simulink model "Pole_placement_track"  (R2023b)
settings: Solver=VariableStepAuto  StartTime=0.0  StopTime=50.0  RelTol=1e-3
values from neighbouring files (symbols this model uses):
  A = double(A)    [Rotational_inverted_pendulum.m]
  A_uns = double(A_uns)    [Rotational_inverted_pendulum.m]
  B = double(B)    [Rotational_inverted_pendulum.m]
  B_uns = double(B_uns)    [Rotational_inverted_pendulum.m]
  C = [1 0 0 0 ... (first row only)    [Rotational_inverted_pendulum.m]
  D = [0 ... (first row only)    [Rotational_inverted_pendulum.m]
  K_pp = place(A,B,P)    [Rotational_inverted_pendulum.m]
  K_pp_uns = place(A_uns,B_uns,P_uns)    [Rotational_inverted_pendulum.m]
  L_kf = lqr(A',C',Q_tilde,R_tilde)'    [Rotational_inverted_pendulum.m]
  L_pp = place(A',C',P_obsv)'    [Rotational_inverted_pendulum.m]
  x1_bar = double(sol.x1)    [Rotational_inverted_pendulum.m]
  x1_bar_uns = x1_bar    [Rotational_inverted_pendulum.m]
  x3_bar = 0    [Rotational_inverted_pendulum.m]
  x3_bar_uns = pi    (= 3.14159265359)    [Rotational_inverted_pendulum.m]
libraries: simulink_extras x10
settings Model: Creator=Mark  LastModifiedBy=Mark

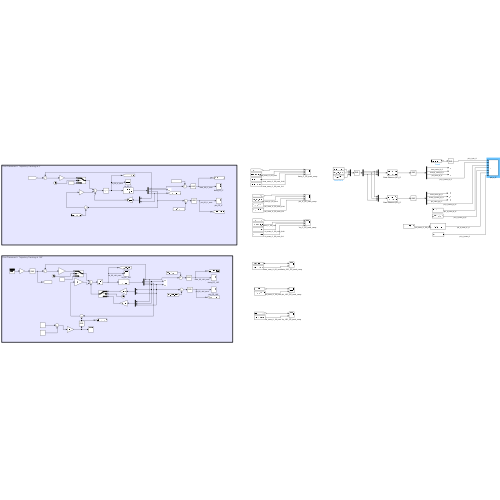
[thumbnail: Simulink's stored preview of the top-level diagram]
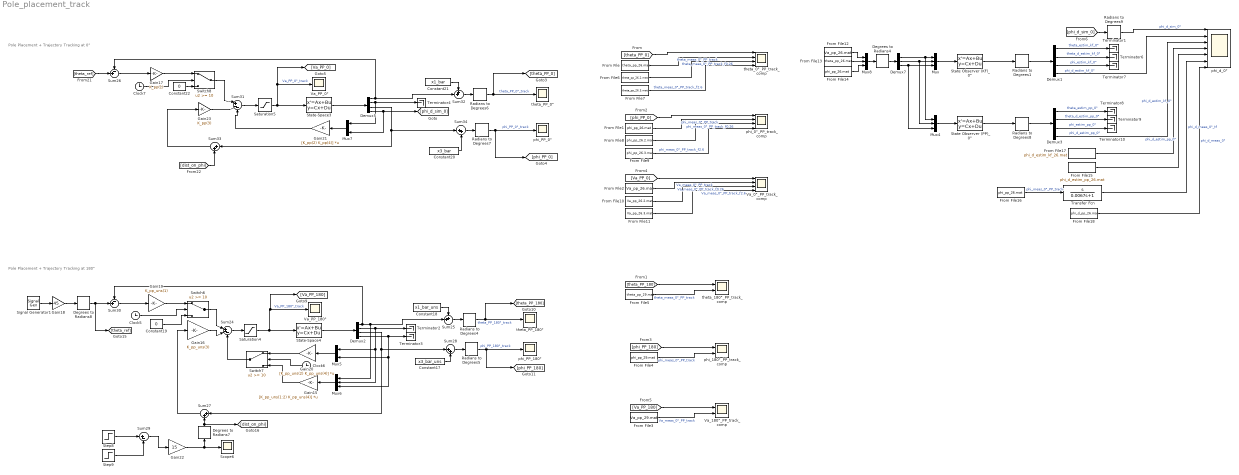
== system Pole_placement_track ==
  note: Pole Placement + Trajectory Tracking at 0°
  note: Pole Placement + Trajectory Tracking at 180°
  Clock5 : Clock
  Clock6 : Clock
  Clock7 : Clock
  Constant17 : Constant  Value=x3_bar_uns
  Constant18 : Constant  Value=x1_bar_uns
  Constant19 : Constant  Value=0
  Constant20 : Constant  Value=x3_bar
  Constant21 : Constant  Value=x1_bar
  Constant22 : Constant  Value=0
  Degrees to Radians4 : simulink_extras/Transformations/Degrees to Radians
  Degrees to Radians7 : simulink_extras/Transformations/Degrees to Radians
  Degrees to Radians8 : simulink_extras/Transformations/Degrees to Radians
  Demux{1..3,5} (4 alike) : Demux
  Demux7 : Demux  Outputs=3
  From File : FromFile  FileName=theta_pp_26.mat  SampleTime=0
  From File1 : FromFile  FileName=phi_pp_26.mat  SampleTime=0
  From File10 : FromFile  FileName=Va_pp_26.2.mat  SampleTime=0
  From File11 : FromFile  FileName=Va_pp_26.3.mat  SampleTime=0
  From File12 : FromFile  FileName=Va_pp_26.mat  SampleTime=0
  From File13 : FromFile  FileName=theta_pp_26.mat  SampleTime=0
  From File14 : FromFile  FileName=phi_pp_26.mat  SampleTime=0
  From File15 : FromFile  FileName=phi_d_estim_pp_26.mat  SampleTime=0
  From File16 : FromFile  FileName=phi_pp_26.mat  SampleTime=0
  From File17 : FromFile  FileName=phi_d_estim_kf_26.mat  SampleTime=0
  From File18 : FromFile  FileName=phi_d_pp_26.mat  SampleTime=0
  From File2 : FromFile  FileName=Va_pp_26.mat  SampleTime=0
  From File3 : FromFile  FileName=Va_pp_29.mat  SampleTime=0
  From File4 : FromFile  FileName=phi_pp_29.mat  SampleTime=0
  From File5 : FromFile  FileName=theta_pp_29.mat  SampleTime=0
  From File6 : FromFile  FileName=theta_pp_26.2.mat  SampleTime=0
  From File7 : FromFile  FileName=theta_pp_26.3.mat  SampleTime=0
  From File8 : FromFile  FileName=phi_pp_26.2.mat  SampleTime=0
  From File9 : FromFile  FileName=phi_pp_26.3.mat  SampleTime=0
  Gain15 : Gain  Gain=[K_pp_uns(1:2) K_pp_uns(4)]  Multiplication=Matrix(K*u) (u vector)
  Gain16 : Gain  Gain=K_pp_uns(3)
  Gain17 : Gain  Gain=K_pp(1)
  Gain18 : Gain  Gain=45
  Gain19 : Gain  Gain=K_pp_uns(1)
  Gain20 : Gain  Gain=[K_pp_uns(2) K_pp_uns(4)]  Multiplication=Matrix(K*u) (u vector)
  Gain21 : Gain  Gain=[K_pp(2) K_pp(4)]  Multiplication=Matrix(K*u) (u vector)
  Gain22 : Gain  Gain=15
  Gain23 : Gain  Gain=K_pp(3)
  Mux{,4,6,8} (4 alike) : Mux  Inputs=3
  Mux5 : Mux  Inputs=2
  Mux7 : Mux  Inputs=2
  Radians to Degrees{1,4..9} (7 alike) : simulink_extras/Transformations/Radians to Degrees
  Saturation4 : Saturate  UpperLimit=10  LowerLimit=-10
  Saturation5 : Saturate  UpperLimit=10  LowerLimit=-10
  Scope6 : Scope
  Signal Generator1 : SignalGenerator  Frequency=2.6
  State Observer (KF)_0° : StateSpace  A=A-L_kf*C  B=[B-L_kf*D L_kf]  C=eye(4)  D=zeros(4,3)  InitialCondition=0  ParameterTunability=Unconstrained
  State Observer (PP)_0° : StateSpace  A=A-L_pp*C  B=[B-L_pp*D L_pp]  C=eye(4)  D=zeros(4,3)  InitialCondition=0
  State-Space3 : StateSpace  A=A  B=B  C=eye(4)  D=zeros(4,1)  InitialCondition=[0 0 0 0]
  State-Space4 : StateSpace  A=A_uns  B=B_uns  C=eye(4)  D=zeros(4,1)  InitialCondition=[0 0 0 0]  ParameterTunability=Optimized
  Step8 : Step  Time=20  SampleTime=0
  Step9 : Step  Time=20.05  SampleTime=0
  Sum24 : Sum  Inputs=|+--
  Sum25 : Sum  Inputs=++|
  Sum26 : Sum  Inputs=-+|
  Sum{27..28,33..34} (4 alike) : Sum  Inputs=|++
  Sum29 : Sum  Inputs=|+-
  Sum30 : Sum  Inputs=-+|
  Sum31 : Sum  Inputs=|+--
  Sum32 : Sum  Inputs=++|
  Switch6 : Switch  Threshold=10  SaturateOnIntegerOverflow=off  InputSameDT=off
  Switch7 : Switch  Threshold=10  SaturateOnIntegerOverflow=off  InputSameDT=off
  Switch8 : Switch  Threshold=10  SaturateOnIntegerOverflow=off  InputSameDT=off
  Terminator{1..4,6..10} (9 alike) : Terminator
  Transfer Fcn : TransferFcn  Numerator=[1 0]  Denominator=[0.0067 1]
  Va_0°_PP_track_comp : Scope  NumInputPorts=4
  Va_180°_PP_track_comp : Scope  NumInputPorts=2
  Va_PP_0° : Scope
  Va_PP_180° : Scope
  phi_0°_PP_track_comp : Scope  NumInputPorts=4
  phi_180°_PP_track_comp : Scope  NumInputPorts=2
  phi_PP_0° : Scope
  phi_PP_180° : Scope
  phi_d_0° : Scope  NumInputPorts=7
  theta_0°_PP_track_comp : Scope  NumInputPorts=4
  theta_180°_PP_track_comp : Scope  NumInputPorts=2
  theta_PP_0° : Scope
  theta_PP_180° : Scope
  wires:
  Switch8/1 -> Sum31/1
  Gain21/1 -> Sum31/3
  Gain23/1 -> Sum31/2
  Sum26/1 -> Gain17/1
  Clock7/1 -> Switch8/2
  Constant21/1 -> Sum32/1
  Demux5/1 -> Sum26/1, Sum32/2
  Sum34/1 -> Radians to Degrees7/1
  Gain17/1 -> Switch8/1
  Sum33/1 -> Gain23/1
  Sum31/1 -> Saturation5/1
  Demux5/3 -> Sum34/1, Sum33/1
  Saturation5/1 -> State-Space3/1, [Va_PP_0], Va_PP_0°/1  "Va_PP_0°_track"
  Mux7/1 -> Gain21/1
  Constant22/1 -> Switch8/3
  Demux5/4 -> [phi_d_sim_0], Mux7/2
  State-Space3/1 -> Demux5/1
  [dist_on_phi] -> Sum33/2
  Sum32/1 -> Radians to Degrees6/1
  Constant20/1 -> Sum34/2
  Demux5/2 -> Mux7/1, Terminator4/1
  [theta_ref] -> Sum26/2
  Radians to Degrees6/1 -> [theta_PP_0], theta_PP_0°/1  "theta_PP_0°_track"
  Radians to Degrees7/1 -> [phi_PP_0], phi_PP_0°/1  "phi_PP_0°_track"
  Sum25/1 -> Radians to Degrees4/1
  Radians to Degrees5/1 -> [phi_PP_180], phi_PP_180°/1  "phi_PP_180°_track"
  Sum28/1 -> Radians to Degrees5/1
  Constant19/1 -> Switch6/3
  Radians to Degrees4/1 -> [theta_PP_180], theta_PP_180°/1  "theta_PP_180°_track"
  Demux2/2 -> Mux5/1, Mux6/2, Terminator2/1
  Degrees to Radians7/1 -> [dist_on_phi], Sum27/2
  Demux2/1 -> Sum30/1, Mux6/1, Sum25/2
  Sum29/1 -> Gain22/1
  Switch7/1 -> Sum24/3
  Constant18/1 -> Sum25/1
  Switch6/1 -> Sum24/1
  Step8/1 -> Sum29/1
  Gain18/1 -> Degrees to Radians8/1
  Clock5/1 -> Switch6/2
  Gain19/1 -> Switch6/1
  Gain22/1 -> Scope6/1, Degrees to Radians7/1
  Degrees to Radians8/1 -> [theta_ref], Sum30/2
  Clock6/1 -> Switch7/2
  Demux2/4 -> Terminator3/1, Mux5/2, Mux6/3
  Sum24/1 -> Saturation4/1
  Step9/1 -> Sum29/2
  Mux6/1 -> Gain15/1
  Mux5/1 -> Gain20/1
  Sum30/1 -> Gain19/1
  Constant17/1 -> Sum28/2
  Saturation4/1 -> State-Space4/1, [Va_PP_180], Va_PP_180°/1  "Va_PP_180°_track"
  State-Space4/1 -> Demux2/1
  Gain16/1 -> Sum24/2
  Demux2/3 -> Sum27/1, Sum28/1
  Sum27/1 -> Gain16/1
  Signal Generator1/1 -> Gain18/1
  Gain15/1 -> Switch7/3
  Gain20/1 -> Switch7/1
  [theta_PP_0] -> theta_0°_PP_track_comp/1
  [phi_PP_0] -> phi_0°_PP_track_comp/1
  [Va_PP_0] -> Va_0°_PP_track_comp/1
  [phi_PP_180] -> phi_180°_PP_track_comp/1
  [Va_PP_180] -> Va_180°_PP_track_comp/1
  [theta_PP_180] -> theta_180°_PP_track_comp/1
  From File5/1 -> theta_180°_PP_track_comp/2  "theta_meas_0°_PP_track"
  From File4/1 -> phi_180°_PP_track_comp/2  "phi_meas_0°_PP_track"
  From File3/1 -> Va_180°_PP_track_comp/2  "Va_meas_0°_PP_track"
  From File2/1 -> Va_0°_PP_track_comp/2  "Va_meas_0°_PP_track"
  From File1/1 -> phi_0°_PP_track_comp/2  "phi_meas_0°_PP_track"
  From File/1 -> theta_0°_PP_track_comp/2  "theta_meas_0°_PP_track"
  From File10/1 -> Va_0°_PP_track_comp/3  "Va_meas_0°_PP_track_f0.26"
  From File11/1 -> Va_0°_PP_track_comp/4  "Va_meas_0°_PP_track_f2.6"
  From File8/1 -> phi_0°_PP_track_comp/3  "phi_meas_0°_PP_track_f0.26"
  From File9/1 -> phi_0°_PP_track_comp/4  "phi_meas_0°_PP_track_f2.6"
  From File6/1 -> theta_0°_PP_track_comp/3  "theta_meas_0°_PP_track_f0.26"
  From File7/1 -> theta_0°_PP_track_comp/4  "theta_meas_0°_PP_track_f2.6"
  Degrees to Radians4/1 -> Demux7/1
  Demux1/3 -> Terminator7/1  "phi_estim_kf_0°"
  From File14/1 -> Mux8/3
  From File15/1 -> phi_d_0°/5  "phi_d_estim_pp_0°"
  From File12/1 -> Mux8/1
  From File13/1 -> Mux8/2
  Mux/1 -> State Observer (KF)_0°/1
  Demux3/4 -> phi_d_0°/3  "phi_d_estim_pp_0°"
  Radians to Degrees8/1 -> Demux3/1
  Mux8/1 -> Degrees to Radians4/1
  State Observer (PP)_0°/1 -> Radians to Degrees8/1
  Demux3/1 -> Terminator8/1  "theta_estim_pp_0°"
  Radians to Degrees1/1 -> Demux1/1
  Demux7/3 -> Mux4/3, Mux/3
  Radians to Degrees9/1 -> phi_d_0°/1  "phi_d_sim_0°"
  Demux1/1 -> Terminator1/1  "theta_estim_kf_0°"
  Demux3/3 -> Terminator10/1  "phi_estim_pp_0°"
  Mux4/1 -> State Observer (PP)_0°/1
  Demux7/2 -> Mux4/2, Mux/2
  State Observer (KF)_0°/1 -> Radians to Degrees1/1
  Demux1/4 -> phi_d_0°/2  "phi_d_estim_kf_0°"
  Demux1/2 -> Terminator6/1  "theta_d_estim_kf_0°"
  [phi_d_sim_0] -> Radians to Degrees9/1
  Demux3/2 -> Terminator9/1  "theta_d_estim_pp_0°"
  Demux7/1 -> Mux4/1, Mux/1
  Transfer Fcn/1 -> phi_d_0°/6  "phi_d_meas_0°_tf"
  From File16/1 -> Transfer Fcn/1  "phi_meas_0°_PP_track"
  From File17/1 -> phi_d_0°/4  "phi_d_estim_kf_0°"
  From File18/1 -> phi_d_0°/7  "phi_d_meas_0°"
